simulink model "rlDQNPFC2"  (R2022b)
settings: Solver=FixedStepAuto  StartTime=0.0  StopTime=Tf  FixedStep=0.001  RelTol=1e-3
StartFcn:
  | %scopes= find_system(bdroot,'BlockType','Scope');
  | %for i = 1:length(scopes)
  | %set_param(scopes{i},'Open','on');
  | %end
values from neighbouring files (symbols this model uses):
  amax_ego = 0.4    [DDPG_1.m]    (also in DQN4.m)
  amin_ego = -0.5    [DDPG_1.m]    (also in DQN4.m)
  Cf = 19000    [DDPG_1.m]    (also in DQN4.m)
  Cr = 33000    [DDPG_1.m]    (also in DQN4.m)
  D_default = 1.5    [DDPG_1.m]    (also in DQN4.m)
  e1_initial = -0.05    [DDPG_1.m]    (also in DQN4.m)
  e2_initial = 0.05    [DDPG_1.m]    (also in DQN4.m)
  Iz = 2875    [DDPG_1.m]    (also in DQN4.m)
  lf = 1.4    [DDPG_1.m]    (also in DQN4.m)
  lr = 1.6    [DDPG_1.m]    (also in DQN4.m)
  m = 1600    [DDPG_1.m]    (also in DQN4.m)
  t_gap = 1.4    [DDPG_1.m]    (also in DQN4.m)
  target = 1    [DDPG_1.m]    (also in DQN4.m = 3)
  tau = 0.5    [DDPG_1.m]    (also in DQN4.m)
  Ts = 0.1    [DDPG_1.m]    (also in DQN4.m)
  umax_ego = 0.2618    [DDPG_1.m]    (also in DQN4.m)
  umin_ego = -0.2618    [DDPG_1.m]    (also in DQN4.m)
  v0_FV1 = 0.5    [DDPG_1.m]    (also in DQN4.m)
  v0_FV2 = 0.5    [DDPG_1.m]    (also in DQN4.m)
  v0_LV = 0.9    [DDPG_1.m]    (also in DQN4.m)
  v_set = 1.5    [DDPG_1.m]    (also in DQN4.m)
  x0_FV1 = 1.5    [DDPG_1.m]    (also in DQN4.m)
  x0_FV2 = 0    [DDPG_1.m]    (also in DQN4.m)
  x0_LV = 3    [DDPG_1.m]    (also in DQN4.m)
undefined symbols (not defined in the file or in its folder): DiscIntNeverNeededParam
libraries: simulink x13, rllib x4
settings Model: Creator=The MathWorks, Inc.  LastModifiedBy=Lenovo
settings SolverCC: AlgebraicLoopSolver=TrustRegion
settings DataIOCC: SaveOutput=off  SignalLogging=off  DSMLogging=off  SaveTime=off  ReturnWorkspaceOutputs=off
settings DebuggingCC: ParameterPrecisionLossMsg=none  UnconnectedInputMsg=warning  UnconnectedOutputMsg=warning  UnconnectedLineMsg=warning  SFMachineParentedDataDiag=warning  ArithmeticOperatorsInVariantConditions=warning
settings ModelReferenceCC: EnableRefExpFcnMdlSchedulingChecks=on
settings SFSimCC: SimUseLocalCustomCode=off
settings RTWCC: RTWUseLocalCustomCode=off

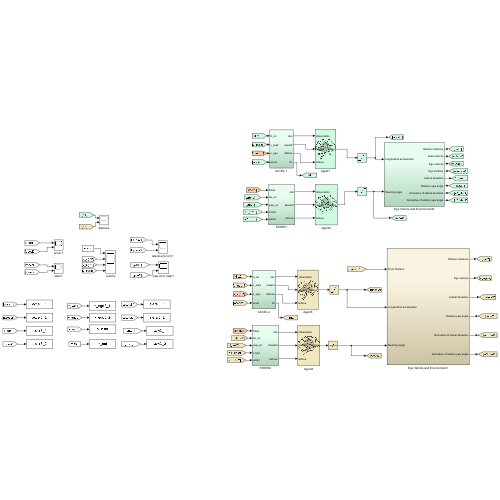
[thumbnail: Simulink's stored preview of the top-level diagram]
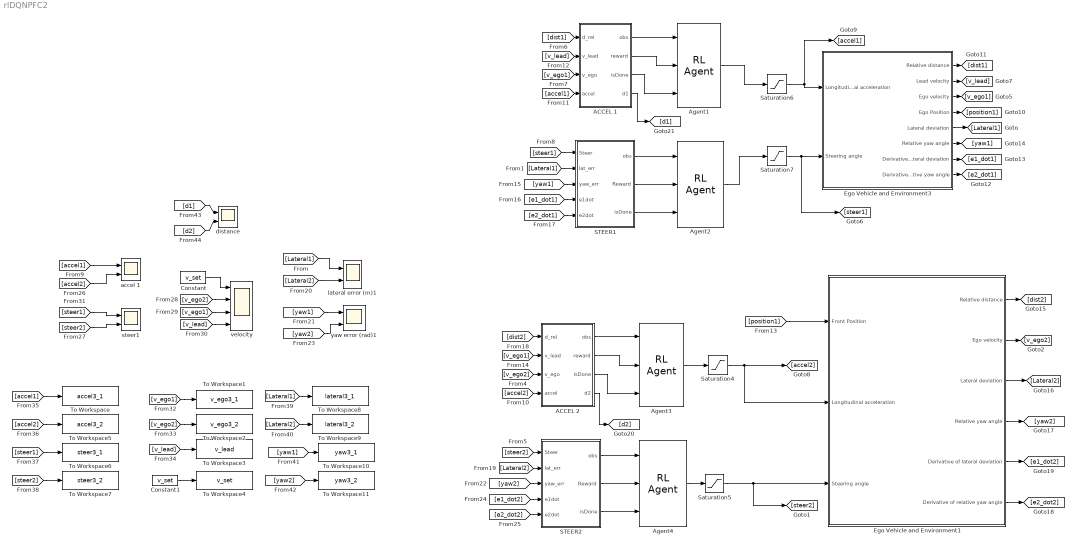
== system rlDQNPFC2 ==
  ACCEL 1 : Subsystem
  ACCEL 2 : Subsystem
  Agent1 : rllib/RL Agent  Agent=agent1  ExternalActionAsInput=off  ProvideLastAction=off  ProvideCumRwd=off  TreatAsDirectFeedthrough=on  UseStrictObservationDataTypes=off
  Agent2 : rllib/RL Agent  Agent=agent2  ExternalActionAsInput=off  ProvideLastAction=off  ProvideCumRwd=off  TreatAsDirectFeedthrough=on  UseStrictObservationDataTypes=off
  Agent3 : rllib/RL Agent  Agent=agent3  ExternalActionAsInput=off  ProvideLastAction=off  ProvideCumRwd=off  TreatAsDirectFeedthrough=on  UseStrictObservationDataTypes=off
  Agent4 : rllib/RL Agent  Agent=agent4  ExternalActionAsInput=off  ProvideLastAction=off  ProvideCumRwd=off  TreatAsDirectFeedthrough=on  UseStrictObservationDataTypes=off
  Constant : Constant  Value=v_set
  Constant1 : Constant  Value=v_set
  Ego Vehicle and Environment1 : Subsystem
  Ego Vehicle and Environment3 : Subsystem
  STEER1 : Subsystem
  STEER2 : Subsystem
  Saturation4 : Saturate  UpperLimit=amax_ego  LowerLimit=amin_ego
  Saturation5 : Saturate  UpperLimit=umax_ego  LowerLimit=umin_ego
  Saturation6 : Saturate  UpperLimit=amax_ego  LowerLimit=amin_ego
  Saturation7 : Saturate  UpperLimit=umax_ego  LowerLimit=umin_ego
  To Workspace : ToWorkspace  VariableName=accel3_1  SampleTime=-1
      settings: Save2DSignal=2-D array (concatenate along first dimension)
  To Workspace1 : ToWorkspace  VariableName=v_ego3_1  SampleTime=-1
      settings: Save2DSignal=2-D array (concatenate along first dimension)
  To Workspace10 : ToWorkspace  VariableName=yaw3_1  SampleTime=-1
      settings: Save2DSignal=2-D array (concatenate along first dimension)
  To Workspace11 : ToWorkspace  VariableName=yaw3_2  SampleTime=-1
      settings: Save2DSignal=2-D array (concatenate along first dimension)
  To Workspace2 : ToWorkspace  VariableName=v_ego3_2  SampleTime=-1
      settings: Save2DSignal=2-D array (concatenate along first dimension)
  To Workspace3 : ToWorkspace  VariableName=v_lead  SampleTime=-1
      settings: Save2DSignal=2-D array (concatenate along first dimension)
  To Workspace4 : ToWorkspace  VariableName=v_set  SampleTime=-1
      settings: Save2DSignal=2-D array (concatenate along first dimension)
  To Workspace5 : ToWorkspace  VariableName=accel3_2  SampleTime=-1
      settings: Save2DSignal=2-D array (concatenate along first dimension)
  To Workspace6 : ToWorkspace  VariableName=steer3_1  SampleTime=-1
      settings: Save2DSignal=2-D array (concatenate along first dimension)
  To Workspace7 : ToWorkspace  VariableName=steer3_2  SampleTime=-1
      settings: Save2DSignal=2-D array (concatenate along first dimension)
  To Workspace8 : ToWorkspace  VariableName=lateral3_1  SampleTime=-1
      settings: Save2DSignal=2-D array (concatenate along first dimension)
  To Workspace9 : ToWorkspace  VariableName=lateral3_2  SampleTime=-1
      settings: Save2DSignal=2-D array (concatenate along first dimension)
  accel 1 : Scope  NumInputPorts=2
  distance : Scope  NumInputPorts=2
  lateral error (m)1 : Scope  NumInputPorts=2
  steer1 : Scope  NumInputPorts=2
  velocity : Scope  NumInputPorts=4
  yaw error (rad)1 : Scope  NumInputPorts=2
  wires:
  [steer1] -> steer1/1
  Ego Vehicle and Environment1/2(Ego velocity) -> [v_ego2]
  [Lateral2] -> STEER2/2(lat_err)
  [v_ego1] -> velocity/3
  Agent3/1 -> Saturation4/1
  Constant/1 -> velocity/1
  [steer2] -> steer1/2
  [accel2] -> accel 1/2
  [accel1] -> accel 1/1
  [yaw2] -> yaw error (rad)1/2
  Ego Vehicle and Environment1/5(Derivative of lateral deviation) -> [e1_dot2]
  Ego Vehicle and Environment1/4(Relative yaw angle) -> [yaw2]
  [yaw2] -> STEER2/3(yaw_err)
  Saturation4/1 -> Ego Vehicle and Environment1/2(Longitudinal acceleration), [accel2]
  [yaw1] -> yaw error (rad)1/1
  [dist2] -> ACCEL 2/1(d_rel)
  [position1] -> Ego Vehicle and Environment1/1(Front Position)
  [v_ego2] -> ACCEL 2/3(v_ego)
  [Lateral2] -> lateral error (m)1/2
  Ego Vehicle and Environment1/6(Derivative of relative yaw angle) -> [e2_dot2]
  [v_ego1] -> ACCEL 2/2(v_lead)
  [steer2] -> STEER2/1(Steer)
  ACCEL 2/1(obs) -> Agent3/1
  ACCEL 2/3(isDone) -> Agent3/3
  STEER2/2(Reward) -> Agent4/2
  STEER2/1(obs) -> Agent4/1
  [v_lead] -> velocity/4
  Ego Vehicle and Environment1/1(Relative distance) -> [dist2]
  [Lateral1] -> lateral error (m)1/1
  [e2_dot2] -> STEER2/5(e2dot)
  Saturation5/1 -> [steer2], Ego Vehicle and Environment1/3(Steering angle)
  STEER2/3(isDone) -> Agent4/3
  Agent4/1 -> Saturation5/1
  Ego Vehicle and Environment1/3(Lateral deviation) -> [Lateral2]
  [accel2] -> ACCEL 2/4(accel)
  [v_ego2] -> velocity/2
  [e1_dot2] -> STEER2/4("e1dot ")
  ACCEL 2/2(reward) -> Agent3/2
  [v_ego1] -> To Workspace1/1
  [v_ego2] -> To Workspace2/1
  [v_lead] -> To Workspace3/1
  Constant1/1 -> To Workspace4/1
  [accel1] -> To Workspace/1
  [accel2] -> To Workspace5/1
  [steer1] -> To Workspace6/1
  [steer2] -> To Workspace7/1
  [Lateral1] -> To Workspace8/1
  [Lateral2] -> To Workspace9/1
  [yaw1] -> To Workspace10/1
  [yaw2] -> To Workspace11/1
  [yaw1] -> STEER1/3(yaw_err)
  [steer1] -> STEER1/1(Steer)
  Ego Vehicle and Environment3/5(Lateral deviation) -> [Lateral1]
  Ego Vehicle and Environment3/6(Relative yaw angle) -> [yaw1]
  Ego Vehicle and Environment3/2(Lead velocity) -> [v_lead]
  [dist1] -> ACCEL 1/1(d_rel)
  Ego Vehicle and Environment3/8(Derivative of relative yaw angle) -> [e2_dot1]
  Ego Vehicle and Environment3/4(Ego Position) -> [position1]
  Saturation7/1 -> Ego Vehicle and Environment3/2(Steering angle), [steer1]
  STEER1/3(isDone) -> Agent2/3
  ACCEL 1/2(reward) -> Agent1/2
  [e2_dot1] -> STEER1/5(e2dot)
  Agent2/1 -> Saturation7/1
  STEER1/2(Reward) -> Agent2/2
  [Lateral1] -> STEER1/2(lat_err)
  [accel1] -> ACCEL 1/4(accel)
  ACCEL 1/3(isDone) -> Agent1/3
  Ego Vehicle and Environment3/3(Ego velocity) -> [v_ego1]
  [e1_dot1] -> STEER1/4("e1dot ")
  Saturation6/1 -> Ego Vehicle and Environment3/1(Longitudinal acceleration), [accel1]
  Ego Vehicle and Environment3/1(Relative distance) -> [dist1]
  STEER1/1(obs) -> Agent2/1
  [v_ego1] -> ACCEL 1/3(v_ego)
  Ego Vehicle and Environment3/7(Derivative of lateral deviation) -> [e1_dot1]
  ACCEL 1/1(obs) -> Agent1/1
  Agent1/1 -> Saturation6/1
  [v_lead] -> ACCEL 1/2(v_lead)
  ACCEL 2/4(d2) -> [d2]
  ACCEL 1/4(d1) -> [d1]
  [d1] -> distance/1
  [d2] -> distance/2

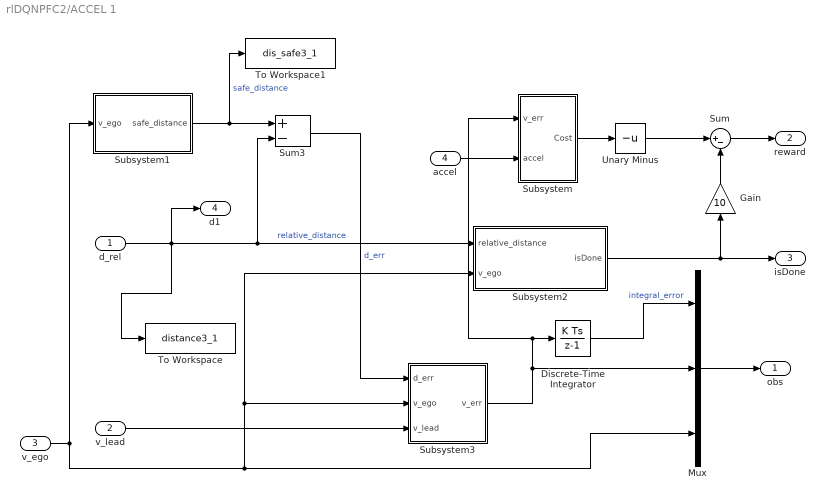
== system rlDQNPFC2/ACCEL 1 ==
  d_rel : Inport
  v_lead : Inport  Port=2
  v_ego : Inport  Port=3
  accel : Inport  Port=4
  Discrete-Time Integrator : DiscreteIntegrator  SampleTime=-1  ICPrevOutput=DiscIntNeverNeededParam  ICPrevScaledInput=DiscIntNeverNeededParam
  Gain : Gain  Gain=10
  Mux : Mux  Inputs=3
  Subsystem : Subsystem
  Subsystem1 : Subsystem
  Subsystem2 : Subsystem
  Subsystem3 : Subsystem
  Sum : Sum  Inputs=|+-
  Sum3 : Sum  Inputs=+-
  To Workspace : ToWorkspace  VariableName=distance3_1  SampleTime=-1
      settings: Save2DSignal=2-D array (concatenate along first dimension)
  To Workspace1 : ToWorkspace  VariableName=dis_safe3_1  SampleTime=-1
      settings: Save2DSignal=2-D array (concatenate along first dimension)
  Unary Minus : UnaryMinus
  obs : Outport  VectorParamsAs1DForOutWhenUnconnected=off
  reward : Outport  Port=2  VectorParamsAs1DForOutWhenUnconnected=off
  isDone : Outport  Port=3  VectorParamsAs1DForOutWhenUnconnected=off
  d1 : Outport  Port=4  VectorParamsAs1DForOutWhenUnconnected=off
  wires:
  v_lead/1 -> Subsystem3/3(v_lead)
  Discrete-Time Integrator/1 -> Mux/1  "integral_error"
  Mux/1 -> obs/1
  v_ego/1 -> Subsystem3/2(v_ego), Subsystem2/2(v_ego), Mux/3, Subsystem1/1(v_ego)
  d_rel/1 -> d1/1, To Workspace/1, Sum3/2, Subsystem2/1(relative_distance)  "relative_distance"
  Subsystem/1(Cost) -> Unary Minus/1
  Sum3/1 -> Subsystem3/1(d_err)  "d_err"
  Subsystem1/1(safe_distance) -> To Workspace1/1, Sum3/1  "safe_distance"
  accel/1 -> Subsystem/2(accel)
  Subsystem3/1(v_err) -> Mux/2, Subsystem/1(v_err), Discrete-Time Integrator/1
  Subsystem2/1(isDone) -> isDone/1, Gain/1
  Unary Minus/1 -> Sum/1
  Gain/1 -> Sum/2
  Sum/1 -> reward/1

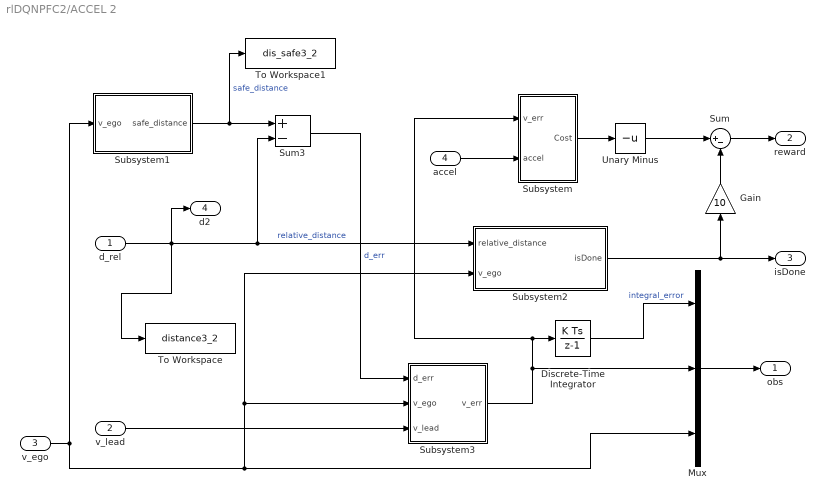
== system rlDQNPFC2/ACCEL 2 ==
  d_rel : Inport
  v_lead : Inport  Port=2
  v_ego : Inport  Port=3
  accel : Inport  Port=4
  Discrete-Time Integrator : DiscreteIntegrator  SampleTime=-1  ICPrevOutput=DiscIntNeverNeededParam  ICPrevScaledInput=DiscIntNeverNeededParam
  Gain : Gain  Gain=10
  Mux : Mux  Inputs=3
  Subsystem : Subsystem
  Subsystem1 : Subsystem
  Subsystem2 : Subsystem
  Subsystem3 : Subsystem
  Sum : Sum  Inputs=|+-
  Sum3 : Sum  Inputs=+-
  To Workspace : ToWorkspace  VariableName=distance3_2  SampleTime=-1
      settings: Save2DSignal=2-D array (concatenate along first dimension)
  To Workspace1 : ToWorkspace  VariableName=dis_safe3_2  SampleTime=-1
      settings: Save2DSignal=2-D array (concatenate along first dimension)
  Unary Minus : UnaryMinus
  obs : Outport  VectorParamsAs1DForOutWhenUnconnected=off
  reward : Outport  Port=2  VectorParamsAs1DForOutWhenUnconnected=off
  isDone : Outport  Port=3  VectorParamsAs1DForOutWhenUnconnected=off
  d2 : Outport  Port=4  VectorParamsAs1DForOutWhenUnconnected=off
  wires:
  Sum/1 -> reward/1
  Gain/1 -> Sum/2
  Unary Minus/1 -> Sum/1
  Subsystem2/1(isDone) -> Gain/1, isDone/1
  Subsystem3/1(v_err) -> Discrete-Time Integrator/1, Subsystem/1(v_err), Mux/2
  accel/1 -> Subsystem/2(accel)
  Subsystem1/1(safe_distance) -> Sum3/1, To Workspace1/1  "safe_distance"
  Sum3/1 -> Subsystem3/1(d_err)  "d_err"
  Subsystem/1(Cost) -> Unary Minus/1
  d_rel/1 -> d2/1, Subsystem2/1(relative_distance), Sum3/2, To Workspace/1  "relative_distance"
  v_ego/1 -> Subsystem1/1(v_ego), Mux/3, Subsystem2/2(v_ego), Subsystem3/2(v_ego)
  Mux/1 -> obs/1
  Discrete-Time Integrator/1 -> Mux/1  "integral_error"
  v_lead/1 -> Subsystem3/3(v_lead)

== system rlDQNPFC2/Ego Vehicle and Environment1 ==
  Front Position : Inport
  Longitudinal acceleration : Inport  Port=2
  Steering angle : Inport  Port=3
  Ego sensor : Subsystem
  Ego vehicle : Subsystem
  Initial ego position : Constant  Value=x0_FV2
  Initial lateral deviation : Constant  Value=e1_initial
  Initial relative yaw angle : Constant  Value=e2_initial
  Sum3 : Sum  Inputs=+-
  curvature1 : Subsystem
  Relative distance : Outport  VectorParamsAs1DForOutWhenUnconnected=off
  Ego velocity : Outport  Port=2  VectorParamsAs1DForOutWhenUnconnected=off
  Lateral deviation : Outport  Port=3  VectorParamsAs1DForOutWhenUnconnected=off
  Relative yaw angle : Outport  Port=4  VectorParamsAs1DForOutWhenUnconnected=off
  Derivative of lateral deviation : Outport  Port=5  VectorParamsAs1DForOutWhenUnconnected=off
  Derivative of relative yaw angle : Outport  Port=6  VectorParamsAs1DForOutWhenUnconnected=off
  wires:
  Ego vehicle/3(Lateral Velocity) -> Ego sensor/2(Lateral velocity)
  Ego vehicle/4(Yaw Rate) -> Ego sensor/3(Yaw rate)
  Longitudinal acceleration/1 -> Ego vehicle/1(Acceleration)  "acceleration"
  Ego sensor/1(Lateral deviation) -> Lateral deviation/1
  Ego vehicle/2(Longitudinal Velocity) -> Ego velocity/1, Ego sensor/1(Longitudinal velocity)
  Steering angle/1 -> Ego vehicle/2(Steering)  "steering"
  Ego sensor/2(Relative yaw angle) -> Relative yaw angle/1
  Initial lateral deviation/1 -> Ego sensor/6(Initial lateral deviation)
  Initial ego position/1 -> Ego vehicle/3(Initial position)
  curvature1/1(curvature) -> Ego sensor/4(Curvature)
  Initial relative yaw angle/1 -> Ego sensor/5(Initial relative yaw angle)
  Front Position/1 -> Sum3/1
  Ego vehicle/1(Position) -> curvature1/1(position), Sum3/2
  Sum3/1 -> Relative distance/1
  Ego sensor/3(e1_dot) -> Derivative of lateral deviation/1
  Ego sensor/4(e2_dot) -> Derivative of relative yaw angle/1

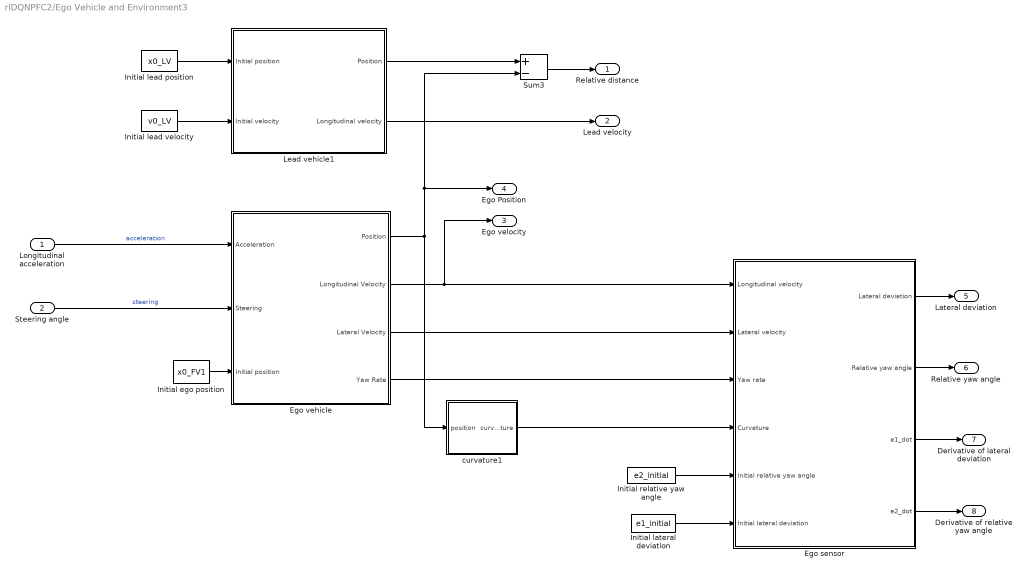
== system rlDQNPFC2/Ego Vehicle and Environment3 ==
  Longitudinal acceleration : Inport
  Steering angle : Inport  Port=2
  Ego sensor : Subsystem
  Ego vehicle : Subsystem
  Initial ego position : Constant  Value=x0_FV1
  Initial lateral deviation : Constant  Value=e1_initial
  Initial lead position : Constant  Value=x0_LV
  Initial lead velocity : Constant  Value=v0_LV
  Initial relative yaw angle : Constant  Value=e2_initial
  Lead vehicle1 : Subsystem
  Sum3 : Sum  Inputs=+-
  curvature1 : Subsystem
  Relative distance : Outport  VectorParamsAs1DForOutWhenUnconnected=off
  Lead velocity : Outport  Port=2  VectorParamsAs1DForOutWhenUnconnected=off
  Ego velocity : Outport  Port=3  VectorParamsAs1DForOutWhenUnconnected=off
  Ego Position : Outport  Port=4
  Lateral deviation : Outport  Port=5  VectorParamsAs1DForOutWhenUnconnected=off
  Relative yaw angle : Outport  Port=6  VectorParamsAs1DForOutWhenUnconnected=off
  Derivative of lateral deviation : Outport  Port=7  VectorParamsAs1DForOutWhenUnconnected=off
  Derivative of relative yaw angle : Outport  Port=8  VectorParamsAs1DForOutWhenUnconnected=off
  wires:
  Ego vehicle/3(Lateral Velocity) -> Ego sensor/2(Lateral velocity)
  Ego vehicle/4(Yaw Rate) -> Ego sensor/3(Yaw rate)
  Longitudinal acceleration/1 -> Ego vehicle/1(Acceleration)  "acceleration"
  Ego sensor/1(Lateral deviation) -> Lateral deviation/1
  Ego vehicle/2(Longitudinal Velocity) -> Ego velocity/1, Ego sensor/1(Longitudinal velocity)
  Steering angle/1 -> Ego vehicle/2(Steering)  "steering"
  Ego sensor/2(Relative yaw angle) -> Relative yaw angle/1
  Initial lateral deviation/1 -> Ego sensor/6(Initial lateral deviation)
  Initial ego position/1 -> Ego vehicle/3(Initial position)
  curvature1/1(curvature) -> Ego sensor/4(Curvature)
  Initial relative yaw angle/1 -> Ego sensor/5(Initial relative yaw angle)
  Initial lead velocity/1 -> Lead vehicle1/2(Initial velocity)
  Initial lead position/1 -> Lead vehicle1/1(Initial position)
  Lead vehicle1/1(Position) -> Sum3/1
  Ego vehicle/1(Position) -> curvature1/1(position), Ego Position/1, Sum3/2
  Sum3/1 -> Relative distance/1
  Lead vehicle1/2(Longitudinal velocity) -> Lead velocity/1
  Ego sensor/3(e1_dot) -> Derivative of lateral deviation/1
  Ego sensor/4(e2_dot) -> Derivative of relative yaw angle/1

== system rlDQNPFC2/STEER1 ==
  Steer : Inport
  lat_err : Inport  Port=2
  yaw_err : Inport  Port=3
  "e1dot " : Inport  Port=4
  e2dot : Inport  Port=5
  Abs : Abs  SaturateOnIntegerOverflow=off
  Compare To Constant : simulink/Logic and Bit Operations/Compare To Constant  relop=>  const=1  OutDataTypeStr=boolean
  Gain : Gain  Gain=10
  Subsystem : Subsystem
  Subsystem1 : Subsystem
  Sum : Sum  Inputs=-+|
  Unary Minus : UnaryMinus
  obs : Outport  VectorParamsAs1DForOutWhenUnconnected=off
  Reward : Outport  Port=2  VectorParamsAs1DForOutWhenUnconnected=off
  isDone : Outport  Port=3  VectorParamsAs1DForOutWhenUnconnected=off
  wires:
  Subsystem/1(Cost) -> Unary Minus/1
  lat_err/1 -> Subsystem1/1(e1), Subsystem/2(e1), Abs/1
  yaw_err/1 -> Subsystem1/2(e2)
  Abs/1 -> Compare To Constant/1
  Subsystem1/1(obs) -> obs/1
  "e1dot "/1 -> Subsystem1/3(e1dot)
  e2dot/1 -> Subsystem1/4(e2dot)
  Steer/1 -> Subsystem/1(steer)
  Compare To Constant/1 -> isDone/1, Gain/1
  Gain/1 -> Sum/1
  Sum/1 -> Reward/1
  Unary Minus/1 -> Sum/2

== system rlDQNPFC2/STEER2 ==
  Steer : Inport
  lat_err : Inport  Port=2
  yaw_err : Inport  Port=3
  "e1dot " : Inport  Port=4
  e2dot : Inport  Port=5
  Abs : Abs  SaturateOnIntegerOverflow=off
  Compare To Constant : simulink/Logic and Bit Operations/Compare To Constant  relop=>  const=1  OutDataTypeStr=boolean
  Gain : Gain  Gain=10
  Subsystem : Subsystem
  Subsystem1 : Subsystem
  Sum : Sum  Inputs=-+|
  Unary Minus : UnaryMinus
  obs : Outport  VectorParamsAs1DForOutWhenUnconnected=off
  Reward : Outport  Port=2  VectorParamsAs1DForOutWhenUnconnected=off
  isDone : Outport  Port=3  VectorParamsAs1DForOutWhenUnconnected=off
  wires:
  Unary Minus/1 -> Sum/2
  Sum/1 -> Reward/1
  Gain/1 -> Sum/1
  Compare To Constant/1 -> Gain/1, isDone/1
  Steer/1 -> Subsystem/1(steer)
  e2dot/1 -> Subsystem1/4(e2dot)
  "e1dot "/1 -> Subsystem1/3(e1dot)
  Subsystem1/1(obs) -> obs/1
  Abs/1 -> Compare To Constant/1
  yaw_err/1 -> Subsystem1/2(e2)
  lat_err/1 -> Abs/1, Subsystem/2(e1), Subsystem1/1(e1)
  Subsystem/1(Cost) -> Unary Minus/1

== system rlDQNPFC2/ACCEL 1/Subsystem ==
  v_err : Inport
  accel : Inport  Port=2
  Compare To Constant : simulink/Logic and Bit Operations/Compare To Constant  relop=<  const=0.09  OutDataTypeStr=boolean
  Gain1 : Gain  Gain=0.1
  Gain2 : Gain  Gain=0.01
  Gain3 : Gain
  Math Function2 : Math  Operator=square  SignedPower=on
  Square : Math  Operator=square  SignedPower=on
  Sum : Sum  Inputs=++-
  Unit Delay : UnitDelay  SampleTime=-1  HasFrameUpgradeWarning=on
  Cost : Outport  VectorParamsAs1DForOutWhenUnconnected=off
  wires:
  v_err/1 -> Square/1
  Math Function2/1 -> Gain1/1
  accel/1 -> Unit Delay/1
  Sum/1 -> Cost/1
  Square/1 -> Compare To Constant/1, Gain2/1
  Unit Delay/1 -> Math Function2/1
  Gain2/1 -> Sum/1
  Gain1/1 -> Sum/2
  Compare To Constant/1 -> Gain3/1
  Gain3/1 -> Sum/3

== system rlDQNPFC2/ACCEL 1/Subsystem1 ==
  v_ego : Inport
  Default Spacing : Constant  Value=D_default  SampleTime=Ts
  Product : Product
  Sum2 : Sum
  Time Gap : Constant  Value=t_gap  SampleTime=Ts
  safe_distance : Outport  VectorParamsAs1DForOutWhenUnconnected=off
  wires:
  Sum2/1 -> safe_distance/1
  Product/1 -> Sum2/2
  Time Gap/1 -> Product/2
  Default Spacing/1 -> Sum2/1
  v_ego/1 -> Product/1

== system rlDQNPFC2/ACCEL 1/Subsystem2 ==
  relative_distance : Inport
  v_ego : Inport  Port=2
  Logical Operator : Logic  Operator=OR  AllPortsSameDT=off  OutDataTypeStr=boolean
  Relative Distance : simulink/Logic and Bit Operations/Compare To Constant  relop=<  const=0  OutDataTypeStr=boolean
  Velocity : simulink/Logic and Bit Operations/Compare To Constant  relop=<  const=0.05  OutDataTypeStr=boolean
  isDone : Outport  VectorParamsAs1DForOutWhenUnconnected=off
  wires:
  Velocity/1 -> Logical Operator/2
  Relative Distance/1 -> Logical Operator/1
  relative_distance/1 -> Relative Distance/1
  Logical Operator/1 -> isDone/1
  v_ego/1 -> Velocity/1

== system rlDQNPFC2/ACCEL 1/Subsystem3 ==
  d_err : Inport
  v_ego : Inport  Port=2
  v_lead : Inport  Port=3
  Constant : Constant  Value=v_set
  Min : MinMax  Inputs=2
  Sum1 : Sum  Inputs=+-
  Switch : Switch  Criteria=u2 > Threshold  SaturateOnIntegerOverflow=off  InputSameDT=off
  v_err : Outport  VectorParamsAs1DForOutWhenUnconnected=off
  wires:
  Sum1/1 -> v_err/1
  v_ego/1 -> Sum1/2
  Switch/1 -> Sum1/1  "v_ref"
  d_err/1 -> Switch/2
  Constant/1 -> Min/2, Switch/3
  Min/1 -> Switch/1
  v_lead/1 -> Min/1

== system rlDQNPFC2/ACCEL 2/Subsystem ==
  v_err : Inport
  accel : Inport  Port=2
  Compare To Constant : simulink/Logic and Bit Operations/Compare To Constant  relop=<  const=0.09  OutDataTypeStr=boolean
  Gain1 : Gain  Gain=0.1
  Gain2 : Gain  Gain=0.01
  Gain3 : Gain
  Math Function2 : Math  Operator=square  SignedPower=on
  Square : Math  Operator=square  SignedPower=on
  Sum : Sum  Inputs=++-
  Unit Delay : UnitDelay  SampleTime=-1  HasFrameUpgradeWarning=on
  Cost : Outport  VectorParamsAs1DForOutWhenUnconnected=off
  wires:
  Gain3/1 -> Sum/3
  Compare To Constant/1 -> Gain3/1
  Gain1/1 -> Sum/2
  Gain2/1 -> Sum/1
  Unit Delay/1 -> Math Function2/1
  Square/1 -> Gain2/1, Compare To Constant/1
  Sum/1 -> Cost/1
  accel/1 -> Unit Delay/1
  Math Function2/1 -> Gain1/1
  v_err/1 -> Square/1

== system rlDQNPFC2/ACCEL 2/Subsystem1 ==
  v_ego : Inport
  Default Spacing : Constant  Value=D_default  SampleTime=Ts
  Product : Product
  Sum2 : Sum
  Time Gap : Constant  Value=t_gap  SampleTime=Ts
  safe_distance : Outport  VectorParamsAs1DForOutWhenUnconnected=off
  wires:
  v_ego/1 -> Product/1
  Default Spacing/1 -> Sum2/1
  Time Gap/1 -> Product/2
  Product/1 -> Sum2/2
  Sum2/1 -> safe_distance/1

== system rlDQNPFC2/ACCEL 2/Subsystem2 ==
  relative_distance : Inport
  v_ego : Inport  Port=2
  Logical Operator : Logic  Operator=OR  AllPortsSameDT=off  OutDataTypeStr=boolean
  Relative Distance : simulink/Logic and Bit Operations/Compare To Constant  relop=<  const=0  OutDataTypeStr=boolean
  Velocity : simulink/Logic and Bit Operations/Compare To Constant  relop=<  const=0.05  OutDataTypeStr=boolean
  isDone : Outport  VectorParamsAs1DForOutWhenUnconnected=off
  wires:
  v_ego/1 -> Velocity/1
  Logical Operator/1 -> isDone/1
  relative_distance/1 -> Relative Distance/1
  Relative Distance/1 -> Logical Operator/1
  Velocity/1 -> Logical Operator/2

== system rlDQNPFC2/ACCEL 2/Subsystem3 ==
  d_err : Inport
  v_ego : Inport  Port=2
  v_lead : Inport  Port=3
  Constant : Constant  Value=v_set
  Min : MinMax  Inputs=2
  Sum1 : Sum  Inputs=+-
  Switch : Switch  Criteria=u2 > Threshold  SaturateOnIntegerOverflow=off  InputSameDT=off
  v_err : Outport  VectorParamsAs1DForOutWhenUnconnected=off
  wires:
  v_lead/1 -> Min/1
  Min/1 -> Switch/1
  Constant/1 -> Switch/3, Min/2
  d_err/1 -> Switch/2
  Switch/1 -> Sum1/1  "v_ref"
  v_ego/1 -> Sum1/2
  Sum1/1 -> v_err/1

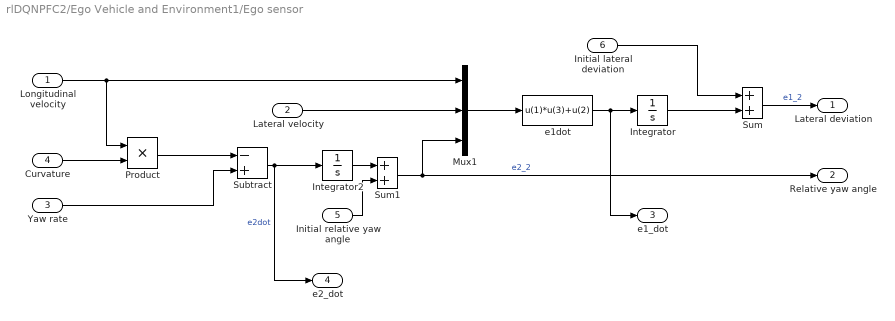
== system rlDQNPFC2/Ego Vehicle and Environment1/Ego sensor ==
  Longitudinal velocity : Inport
  Lateral velocity : Inport  Port=2
  Yaw rate : Inport  Port=3
  Curvature : Inport  Port=4
  Initial relative yaw angle : Inport  Port=5
  Initial lateral deviation : Inport  Port=6
  Integrator : Integrator
  Integrator2 : Integrator
  Mux1 : Mux  Inputs=[1 1 1]
  Product : Product
  Subtract : Sum  Inputs=-+
  Sum : Sum
  Sum1 : Sum
  e1dot : Fcn  Expr=u(1)*u(3)+u(2)
  Lateral deviation : Outport  VectorParamsAs1DForOutWhenUnconnected=off
  Relative yaw angle : Outport  Port=2  VectorParamsAs1DForOutWhenUnconnected=off
  e1_dot : Outport  Port=3  VectorParamsAs1DForOutWhenUnconnected=off
  e2_dot : Outport  Port=4  VectorParamsAs1DForOutWhenUnconnected=off
  wires:
  Curvature/1 -> Product/2
  Sum1/1 -> Mux1/3, Relative yaw angle/1  "e2_2"
  Mux1/1 -> e1dot/1
  Initial lateral deviation/1 -> Sum/1
  e1dot/1 -> e1_dot/1, Integrator/1
  Integrator/1 -> Sum/2
  Longitudinal velocity/1 -> Product/1, Mux1/1
  Lateral velocity/1 -> Mux1/2
  Sum/1 -> Lateral deviation/1  "e1_2"
  Integrator2/1 -> Sum1/1
  Initial relative yaw angle/1 -> Sum1/2
  Product/1 -> Subtract/1
  Yaw rate/1 -> Subtract/2
  Subtract/1 -> e2_dot/1, Integrator2/1  "e2dot"

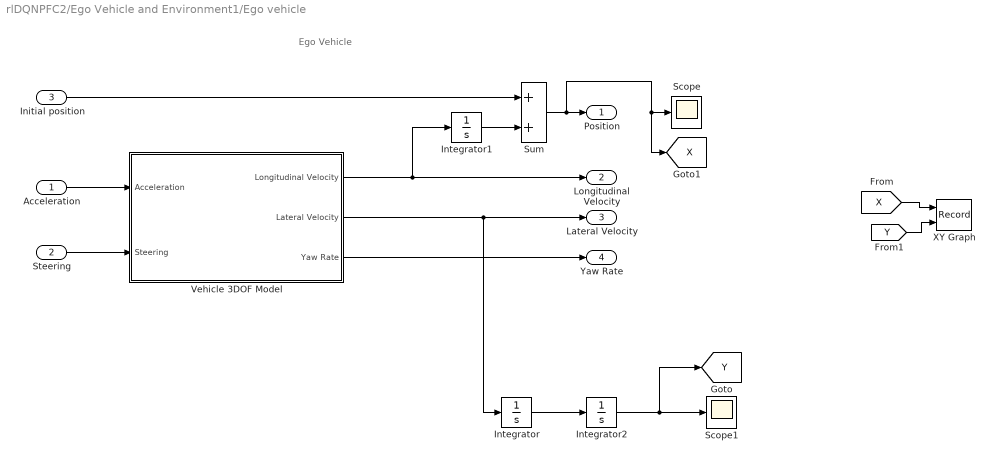
== system rlDQNPFC2/Ego Vehicle and Environment1/Ego vehicle ==
  note: Ego Vehicle
  Acceleration : Inport
  Steering : Inport  Port=2
  Initial position : Inport  Port=3
  Integrator : Integrator
  Integrator1 : Integrator
  Integrator2 : Integrator
  Scope : Scope
  Scope1 : Scope
  Sum : Sum
  Vehicle 3DOF Model : Subsystem
  XY Graph : Record  FileSettingsInternal="{\"entries\":[{\"content\":{\"excelSettings\":{\"content\":{},\"type\":\"Streamout.ExcelSettings\"}},\"type\":\"Streamout.FileSettingStorage\",\"uuid\":\"926f95c6-678a-42c3-81c2-7d91716961ee\"}],\"packageUris\":[\"http://schema.mathworks.com/mf0/streamout_blocks/R2020a\"],\"version\":\"1.0\"}"  Layout=[1 1]  SignalsInternal="{\"entries\":[{\"content\":{\"signals\":[{\"content\":{\"blockPath\":[\"rlDQNPFC2/Ego Vehicle and Environment1/Ego vehicle/XY Graph\"],\"channel\":[],\"dimensions\":[1],\"domain\":\"rlDQNPFC2/Ego Vehicle and Environment1/Ego vehicle/XY Graph\",\"lineColor\":\"#139fff\",\"plots\":[],\"port\":1,\"sid\":[],\"signalID\":2481,\"signalName\":\"From\"},\"type\":\"RecordBlkView.Signal\",\"uuid\":\"ba51d43c-8927-4175-b2ca-93bf3e4e2194\"},{\"content\":{\"blockPath\":[\"rlDQNPFC2/Ego Vehicle and Environment1/Ego vehicle/XY Graph\"],\"channel\":[],\"dimensions\":[1],\"domain\":\"rlDQNPFC2/Ego Vehicle and Environment1/Ego vehicle/XY Graph\",\"lineColor\":\"#ff6929\",\"plots\":[],\"port\":2,\"sid\":[],\"signalID\":2484,\"signalName\":\"From1\"},\"type\":\"RecordBlkView.Signal\",\"uuid\":\"ffd6dc64-998e-4497-b7fe-adbc949d6770\"}]},\"type\":\"RecordBlkView.InputSignals\",\"uuid\":\"4b290cac-6114-4463-9ac7-c2a0d02c0e46\"}],\"packageUris\":[\"http://schema.mathworks.com/mf0/streamout_blocks/R2020a\"],\"version\":\"1.0\"}"  CompatibilityTag=XY
  Position : Outport  VectorParamsAs1DForOutWhenUnconnected=off
  Longitudinal Velocity : Outport  Port=2  VectorParamsAs1DForOutWhenUnconnected=off
  Lateral Velocity : Outport  Port=3  VectorParamsAs1DForOutWhenUnconnected=off
  Yaw Rate : Outport  Port=4  VectorParamsAs1DForOutWhenUnconnected=off
  tag scope: X=global, Y=global
  wires:
  Integrator1/1 -> Sum/2
  Initial position/1 -> Sum/1
  Acceleration/1 -> Vehicle 3DOF Model/1(Acceleration)
  Steering/1 -> Vehicle 3DOF Model/2(Steering)
  Vehicle 3DOF Model/3(Yaw Rate) -> Yaw Rate/1
  Vehicle 3DOF Model/1(Longitudinal Velocity) -> Longitudinal Velocity/1, Integrator1/1
  Sum/1 -> [X], Scope/1, Position/1
  Vehicle 3DOF Model/2(Lateral Velocity) -> Integrator/1, Lateral Velocity/1
  Integrator/1 -> Integrator2/1
  Integrator2/1 -> [Y], Scope1/1
  [X] -> XY Graph/1
  [Y] -> XY Graph/2

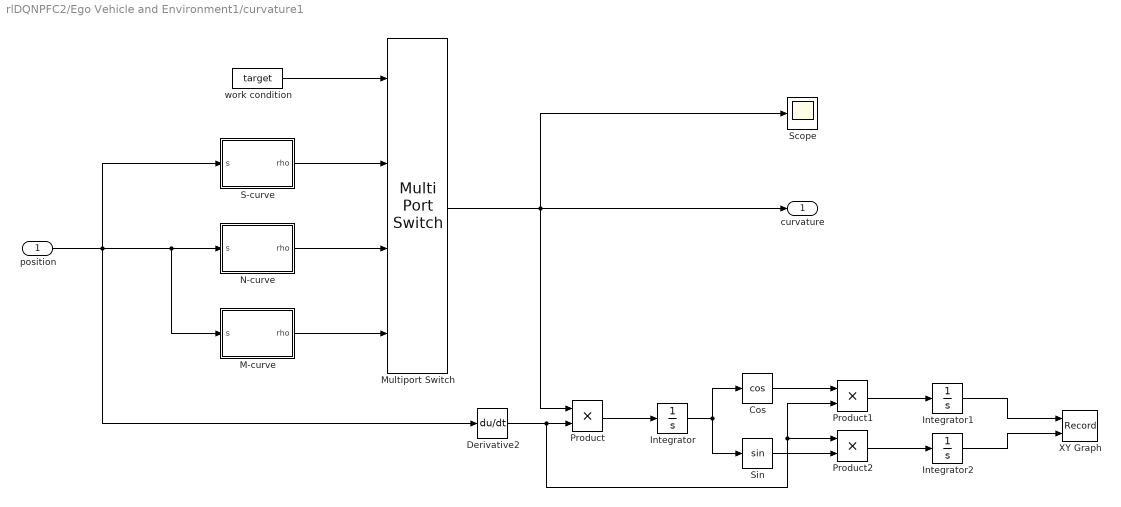
== system rlDQNPFC2/Ego Vehicle and Environment1/curvature1 ==
  position : Inport
  Cos : Trigonometry  Operator=cos
  Derivative2 : Derivative
  Integrator : Integrator
  Integrator1 : Integrator
  Integrator2 : Integrator
  M-curve : MATLAB Function  TreatAsAtomicUnit=on
  Multiport Switch : MultiPortSwitch  SaturateOnIntegerOverflow=off  InputSameDT=off
  N-curve : MATLAB Function  TreatAsAtomicUnit=on
  Product : Product
  Product1 : Product
  Product2 : Product
  S-curve : MATLAB Function  TreatAsAtomicUnit=on
  Scope : Scope
  Sin : Trigonometry
  XY Graph : Record  FileSettingsInternal="{\"entries\":[{\"content\":{\"excelSettings\":{\"content\":{},\"type\":\"Streamout.ExcelSettings\"}},\"type\":\"Streamout.FileSettingStorage\",\"uuid\":\"a88f7f64-6dc8-4fad-b474-f6daca30f32e\"}],\"packageUris\":[\"http://schema.mathworks.com/mf0/streamout_blocks/R2020a\"],\"version\":\"1.0\"}"  Layout=[1 1]  SignalsInternal="{\"entries\":[{\"content\":{\"signals\":[{\"content\":{\"blockPath\":[\"rlDQNPFC2/Ego Vehicle and Environment1/curvature1/XY Graph\"],\"channel\":[],\"dimensions\":[1],\"domain\":\"rlDQNPFC2/Ego Vehicle and Environment1/curvature1/XY Graph\",\"lineColor\":\"#b746ff\",\"plots\":[],\"port\":1,\"sid\":[],\"signalID\":2473,\"signalName\":\"Integrator1\"},\"type\":\"RecordBlkView.Signal\",\"uuid\":\"be24a98a-5aff-47ce-ad63-fb56a4aae694\"},{\"content\":{\"blockPath\":[\"rlDQNPFC2/Ego Vehicle and Environment1/curvature1/XY Graph\"],\"channel\":[],\"dimensions\":[1],\"domain\":\"rlDQNPFC2/Ego Vehicle and Environment1/curvature1/XY Graph\",\"lineColor\":\"#64d413\",\"plots\":[],\"port\":2,\"sid\":[],\"signalID\":2476,\"signalName\":\"Integrator2\"},\"type\":\"RecordBlkView.Signal\",\"uuid\":\"fdd17382-7340-4eb7-bf1d-fe8a0e01edb1\"}]},\"type\":\"RecordBlkView.InputSignals\",\"uuid\":\"159e895c-7bf5-4838-b84f-f7ecce4a2c9b\"}],\"packageUris\":[\"http://schema.mathworks.com/mf0/streamout_blocks/R2020a\"],\"version\":\"1.0\"}"  VisualizationBindings="{\"xyplotplugin\":{\"info\":[{\"series\":[],\"subplotID\":1}]}}"  CompatibilityTag=XY
  work condition : Constant  Value=target
  curvature : Outport
  wires:
  Integrator1/1 -> XY Graph/1
  Integrator2/1 -> XY Graph/2
  Integrator/1 -> Cos/1, Sin/1
  Derivative2/1 -> Product1/2, Product2/1, Product/2
  Product/1 -> Integrator/1
  Product2/1 -> Integrator2/1
  Sin/1 -> Product2/2
  Product1/1 -> Integrator1/1
  Cos/1 -> Product1/1
  position/1 -> S-curve/1(s), Derivative2/1, M-curve/1(s), N-curve/1(s)
  Multiport Switch/1 -> Product/1, curvature/1, Scope/1
  S-curve/1(rho) -> Multiport Switch/2
  N-curve/1(rho) -> Multiport Switch/3
  work condition/1 -> Multiport Switch/1
  M-curve/1(rho) -> Multiport Switch/4

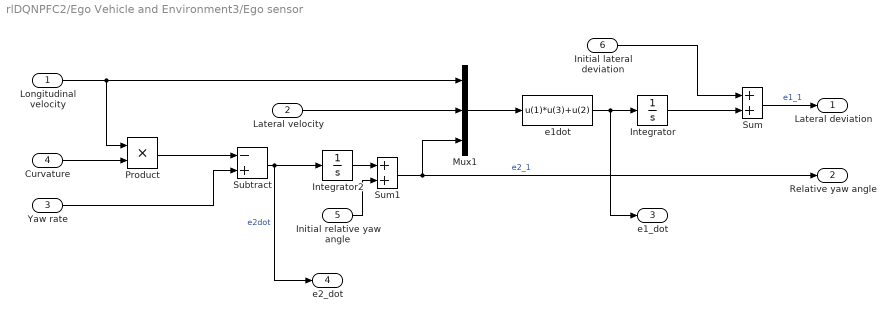
== system rlDQNPFC2/Ego Vehicle and Environment3/Ego sensor ==
  Longitudinal velocity : Inport
  Lateral velocity : Inport  Port=2
  Yaw rate : Inport  Port=3
  Curvature : Inport  Port=4
  Initial relative yaw angle : Inport  Port=5
  Initial lateral deviation : Inport  Port=6
  Integrator : Integrator
  Integrator2 : Integrator
  Mux1 : Mux  Inputs=[1 1 1]
  Product : Product
  Subtract : Sum  Inputs=-+
  Sum : Sum
  Sum1 : Sum
  e1dot : Fcn  Expr=u(1)*u(3)+u(2)
  Lateral deviation : Outport  VectorParamsAs1DForOutWhenUnconnected=off
  Relative yaw angle : Outport  Port=2  VectorParamsAs1DForOutWhenUnconnected=off
  e1_dot : Outport  Port=3  VectorParamsAs1DForOutWhenUnconnected=off
  e2_dot : Outport  Port=4  VectorParamsAs1DForOutWhenUnconnected=off
  wires:
  Curvature/1 -> Product/2
  Sum1/1 -> Mux1/3, Relative yaw angle/1  "e2_1"
  Mux1/1 -> e1dot/1
  Initial lateral deviation/1 -> Sum/1
  e1dot/1 -> e1_dot/1, Integrator/1
  Integrator/1 -> Sum/2
  Longitudinal velocity/1 -> Product/1, Mux1/1
  Lateral velocity/1 -> Mux1/2
  Sum/1 -> Lateral deviation/1  "e1_1"
  Integrator2/1 -> Sum1/1
  Initial relative yaw angle/1 -> Sum1/2
  Product/1 -> Subtract/1
  Yaw rate/1 -> Subtract/2
  Subtract/1 -> e2_dot/1, Integrator2/1  "e2dot"

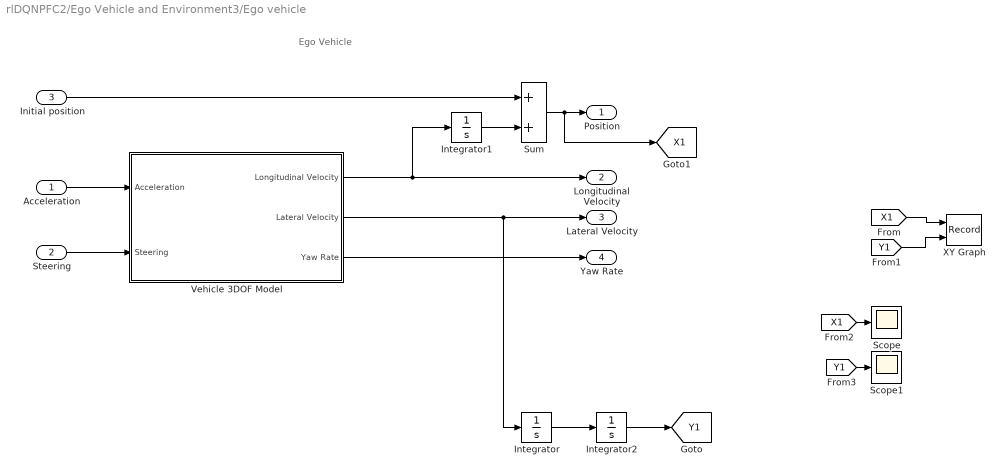
== system rlDQNPFC2/Ego Vehicle and Environment3/Ego vehicle ==
  note: Ego Vehicle
  Acceleration : Inport
  Steering : Inport  Port=2
  Initial position : Inport  Port=3
  Integrator : Integrator
  Integrator1 : Integrator
  Integrator2 : Integrator
  Scope : Scope
  Scope1 : Scope
  Sum : Sum
  Vehicle 3DOF Model : Subsystem
  XY Graph : Record  FileSettingsInternal="{\"entries\":[{\"content\":{\"excelSettings\":{\"content\":{},\"type\":\"Streamout.ExcelSettings\"}},\"type\":\"Streamout.FileSettingStorage\",\"uuid\":\"b77e72f0-3780-4628-8c22-82802707b8c2\"}],\"packageUris\":[\"http://schema.mathworks.com/mf0/streamout_blocks/R2020a\"],\"version\":\"1.0\"}"  Layout=[1 1]  SignalsInternal="{\"entries\":[{\"content\":{\"signals\":[{\"content\":{\"blockPath\":[\"rlDQNPFC2/Ego Vehicle and Environment3/Ego vehicle/XY Graph\"],\"channel\":[],\"dimensions\":[1],\"domain\":\"rlDQNPFC2/Ego Vehicle and Environment3/Ego vehicle/XY Graph\",\"lineColor\":\"#ff13a6\",\"plots\":[],\"port\":1,\"sid\":[],\"signalID\":2465,\"signalName\":\"From\"},\"type\":\"RecordBlkView.Signal\",\"uuid\":\"8eb38749-574b-4766-8d65-6162ff162a27\"},{\"content\":{\"blockPath\":[\"rlDQNPFC2/Ego Vehicle and Environment3/Ego vehicle/XY Graph\"],\"channel\":[],\"dimensions\":[1],\"domain\":\"rlDQNPFC2/Ego Vehicle and Environment3/Ego vehicle/XY Graph\",\"lineColor\":\"#fe330a\",\"plots\":[],\"port\":2,\"sid\":[],\"signalID\":2468,\"signalName\":\"From1\"},\"type\":\"RecordBlkView.Signal\",\"uuid\":\"504250fa-d97e-40d2-a22b-9ec899ac93c3\"}]},\"type\":\"RecordBlkView.InputSignals\",\"uuid\":\"abb257bf-f213-4b71-872b-4d0fb6c25c0d\"}],\"packageUris\":[\"http://schema.mathworks.com/mf0/streamout_blocks/R2020a\"],\"version\":\"1.0\"}"  VisualizationBindings="{\"sparklinesplugin\":{\"info\":[{\"bindingParametersList\":[],\"subplotID\":1}]}}"  CompatibilityTag=XY
  Position : Outport  VectorParamsAs1DForOutWhenUnconnected=off
  Longitudinal Velocity : Outport  Port=2  VectorParamsAs1DForOutWhenUnconnected=off
  Lateral Velocity : Outport  Port=3  VectorParamsAs1DForOutWhenUnconnected=off
  Yaw Rate : Outport  Port=4  VectorParamsAs1DForOutWhenUnconnected=off
  tag scope: X1=global, Y1=global
  wires:
  Integrator1/1 -> Sum/2
  Initial position/1 -> Sum/1
  Acceleration/1 -> Vehicle 3DOF Model/1(Acceleration)
  Steering/1 -> Vehicle 3DOF Model/2(Steering)
  Vehicle 3DOF Model/3(Yaw Rate) -> Yaw Rate/1
  Vehicle 3DOF Model/1(Longitudinal Velocity) -> Longitudinal Velocity/1, Integrator1/1
  Vehicle 3DOF Model/2(Lateral Velocity) -> Integrator/1, Lateral Velocity/1
  Sum/1 -> [X1], Position/1
  Integrator2/1 -> [Y1]
  Integrator/1 -> Integrator2/1
  [X1] -> XY Graph/1
  [Y1] -> XY Graph/2
  [X1] -> Scope/1
  [Y1] -> Scope1/1

== system rlDQNPFC2/Ego Vehicle and Environment3/Lead vehicle1 ==
  Initial position : Inport
  Initial velocity : Inport  Port=2
  Constant : Constant  Value=target
  Integrator : Integrator
  Integrator1 : Integrator
  Multiport Switch1 : MultiPortSwitch  SaturateOnIntegerOverflow=off  InputSameDT=off
  Sine1 : Sin  Amplitude=0.05  Frequency=2*pi/60  SampleTime=Ts
  Sum : Sum
  Sum1 : Sum
  Transfer Fcn : TransferFcn  Denominator=[0.6 1]
  a_LV : Scope
  ramp1 : Subsystem
  step1 : Subsystem
  Position : Outport  VectorParamsAs1DForOutWhenUnconnected=off
  Longitudinal velocity : Outport  Port=2  VectorParamsAs1DForOutWhenUnconnected=off
  wires:
  Transfer Fcn/1 -> Sum1/1
  Initial velocity/1 -> Sum1/2
  Sum/1 -> Position/1
  Integrator/1 -> Transfer Fcn/1
  Sum1/1 -> Integrator1/1, Longitudinal velocity/1
  Initial position/1 -> Sum/1
  Integrator1/1 -> Sum/2
  Sine1/1 -> Multiport Switch1/3  "a_LV"
  ramp1/1(Out1) -> Multiport Switch1/2
  step1/1(a_LV) -> Multiport Switch1/4
  Multiport Switch1/1 -> a_LV/1, Integrator/1  "a_LV"
  Constant/1 -> Multiport Switch1/1

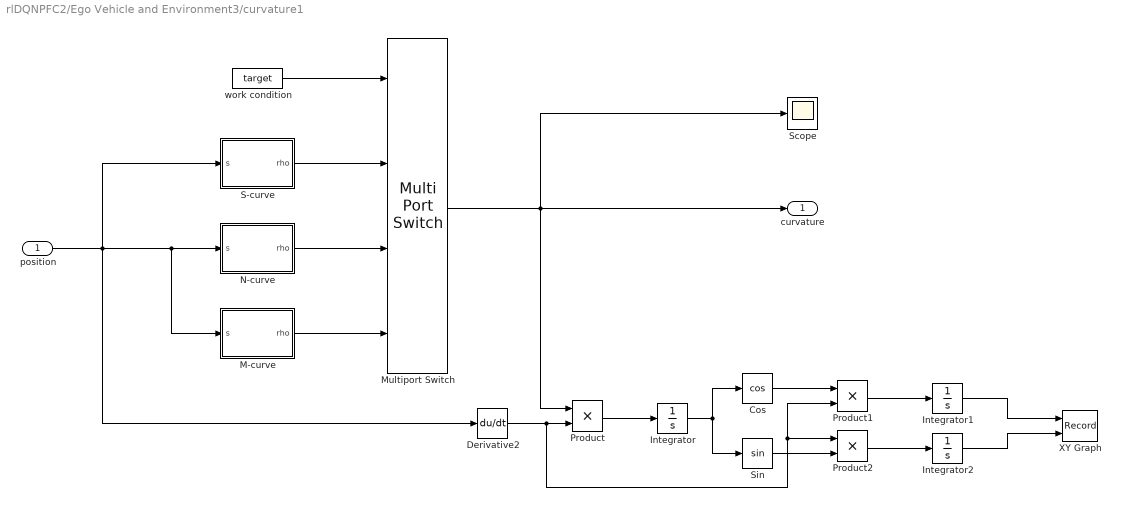
== system rlDQNPFC2/Ego Vehicle and Environment3/curvature1 ==
  position : Inport
  Cos : Trigonometry  Operator=cos
  Derivative2 : Derivative
  Integrator : Integrator
  Integrator1 : Integrator
  Integrator2 : Integrator
  M-curve : MATLAB Function  TreatAsAtomicUnit=on
  Multiport Switch : MultiPortSwitch  SaturateOnIntegerOverflow=off  InputSameDT=off
  N-curve : MATLAB Function  TreatAsAtomicUnit=on
  Product : Product
  Product1 : Product
  Product2 : Product
  S-curve : MATLAB Function  TreatAsAtomicUnit=on
  Scope : Scope
  Sin : Trigonometry
  XY Graph : Record  FileSettingsInternal="{\"entries\":[{\"content\":{\"excelSettings\":{\"content\":{},\"type\":\"Streamout.ExcelSettings\"}},\"type\":\"Streamout.FileSettingStorage\",\"uuid\":\"914a34ab-5b3d-44af-9583-0c2c75f12d06\"}],\"packageUris\":[\"http://schema.mathworks.com/mf0/streamout_blocks/R2020a\"],\"version\":\"1.0\"}"  Layout=[1 1]  SignalsInternal="{\"entries\":[{\"content\":{\"signals\":[{\"content\":{\"blockPath\":[\"rlDQNPFC2/Ego Vehicle and Environment3/curvature1/XY Graph\"],\"channel\":[],\"dimensions\":[1],\"domain\":\"rlDQNPFC2/Ego Vehicle and Environment3/curvature1/XY Graph\",\"lineColor\":\"#22b573\",\"plots\":[],\"port\":1,\"sid\":[],\"signalID\":2457,\"signalName\":\"Integrator1\"},\"type\":\"RecordBlkView.Signal\",\"uuid\":\"51aef201-808c-4e46-946c-300a715014d8\"},{\"content\":{\"blockPath\":[\"rlDQNPFC2/Ego Vehicle and Environment3/curvature1/XY Graph\"],\"channel\":[],\"dimensions\":[1],\"domain\":\"rlDQNPFC2/Ego Vehicle and Environment3/curvature1/XY Graph\",\"lineColor\":\"#0072bd\",\"plots\":[],\"port\":2,\"sid\":[],\"signalID\":2460,\"signalName\":\"Integrator2\"},\"type\":\"RecordBlkView.Signal\",\"uuid\":\"bebfd558-065c-412e-a7bd-9710741a958a\"}]},\"type\":\"RecordBlkView.InputSignals\",\"uuid\":\"30e76bc6-5273-4dec-8796-09d7f0daaaf9\"}],\"packageUris\":[\"http://schema.mathworks.com/mf0/streamout_blocks/R2020a\"],\"version\":\"1.0\"}"  VisualizationBindings="{\"xyplotplugin\":{\"info\":[{\"series\":[],\"subplotID\":1}]}}"  CompatibilityTag=XY
  work condition : Constant  Value=target
  curvature : Outport
  wires:
  Integrator1/1 -> XY Graph/1
  Integrator2/1 -> XY Graph/2
  Integrator/1 -> Cos/1, Sin/1
  Derivative2/1 -> Product1/2, Product2/1, Product/2
  Product/1 -> Integrator/1
  Product2/1 -> Integrator2/1
  Sin/1 -> Product2/2
  Product1/1 -> Integrator1/1
  Cos/1 -> Product1/1
  position/1 -> S-curve/1(s), Derivative2/1, M-curve/1(s), N-curve/1(s)
  Multiport Switch/1 -> Product/1, curvature/1, Scope/1
  S-curve/1(rho) -> Multiport Switch/2
  N-curve/1(rho) -> Multiport Switch/3
  work condition/1 -> Multiport Switch/1
  M-curve/1(rho) -> Multiport Switch/4

== system rlDQNPFC2/STEER1/Subsystem ==
  steer : Inport
  e1 : Inport  Port=2
  Compare To Constant1 : simulink/Logic and Bit Operations/Compare To Constant  relop=<  const=0.01  OutDataTypeStr=boolean
  Gain : Gain  Gain=0.1
  Gain2 : Gain  Gain=0.5
  Gain5 : Gain  Gain=2
  Square : Math  Operator=square  SignedPower=on
  Square2 : Math  Operator=square  SignedPower=on
  Sum1 : Sum  Inputs=-++
  Unit Delay : UnitDelay  SampleTime=-1  HasFrameUpgradeWarning=on
  Cost : Outport  VectorParamsAs1DForOutWhenUnconnected=off
  wires:
  e1/1 -> Square/1
  Sum1/1 -> Cost/1
  Gain/1 -> Sum1/2
  steer/1 -> Unit Delay/1
  Square2/1 -> Gain2/1
  Gain2/1 -> Sum1/3
  Unit Delay/1 -> Square2/1
  Compare To Constant1/1 -> Gain5/1
  Square/1 -> Compare To Constant1/1, Gain/1
  Gain5/1 -> Sum1/1

== system rlDQNPFC2/STEER1/Subsystem1 ==
  e1 : Inport
  e2 : Inport  Port=2
  e1dot : Inport  Port=3
  e2dot : Inport  Port=4
  Discrete-Time Integrator : DiscreteIntegrator  SampleTime=-1  ICPrevOutput=DiscIntNeverNeededParam  ICPrevScaledInput=DiscIntNeverNeededParam
  Discrete-Time Integrator1 : DiscreteIntegrator  SampleTime=-1  ICPrevOutput=DiscIntNeverNeededParam  ICPrevScaledInput=DiscIntNeverNeededParam
  Mux : Mux  Inputs=6
  obs : Outport  VectorParamsAs1DForOutWhenUnconnected=off
  wires:
  e1/1 -> Mux/2, Discrete-Time Integrator1/1
  Mux/1 -> obs/1
  Discrete-Time Integrator1/1 -> Mux/1  "integral_error"
  e2/1 -> Mux/4, Discrete-Time Integrator/1
  Discrete-Time Integrator/1 -> Mux/3  "integral_error"
  e1dot/1 -> Mux/5
  e2dot/1 -> Mux/6

== system rlDQNPFC2/STEER2/Subsystem ==
  steer : Inport
  e1 : Inport  Port=2
  Compare To Constant1 : simulink/Logic and Bit Operations/Compare To Constant  relop=<  const=0.01  OutDataTypeStr=boolean
  Gain : Gain  Gain=0.1
  Gain2 : Gain  Gain=0.5
  Gain5 : Gain  Gain=2
  Square : Math  Operator=square  SignedPower=on
  Square2 : Math  Operator=square  SignedPower=on
  Sum1 : Sum  Inputs=-++
  Unit Delay : UnitDelay  SampleTime=-1  HasFrameUpgradeWarning=on
  Cost : Outport  VectorParamsAs1DForOutWhenUnconnected=off
  wires:
  Gain5/1 -> Sum1/1
  Square/1 -> Gain/1, Compare To Constant1/1
  Compare To Constant1/1 -> Gain5/1
  Unit Delay/1 -> Square2/1
  Gain2/1 -> Sum1/3
  Square2/1 -> Gain2/1
  steer/1 -> Unit Delay/1
  Gain/1 -> Sum1/2
  Sum1/1 -> Cost/1
  e1/1 -> Square/1

== system rlDQNPFC2/STEER2/Subsystem1 ==
  e1 : Inport
  e2 : Inport  Port=2
  e1dot : Inport  Port=3
  e2dot : Inport  Port=4
  Discrete-Time Integrator : DiscreteIntegrator  SampleTime=-1  ICPrevOutput=DiscIntNeverNeededParam  ICPrevScaledInput=DiscIntNeverNeededParam
  Discrete-Time Integrator1 : DiscreteIntegrator  SampleTime=-1  ICPrevOutput=DiscIntNeverNeededParam  ICPrevScaledInput=DiscIntNeverNeededParam
  Mux : Mux  Inputs=6
  obs : Outport  VectorParamsAs1DForOutWhenUnconnected=off
  wires:
  e2dot/1 -> Mux/6
  e1dot/1 -> Mux/5
  Discrete-Time Integrator/1 -> Mux/3  "integral_error"
  e2/1 -> Discrete-Time Integrator/1, Mux/4
  Discrete-Time Integrator1/1 -> Mux/1  "integral_error"
  Mux/1 -> obs/1
  e1/1 -> Discrete-Time Integrator1/1, Mux/2

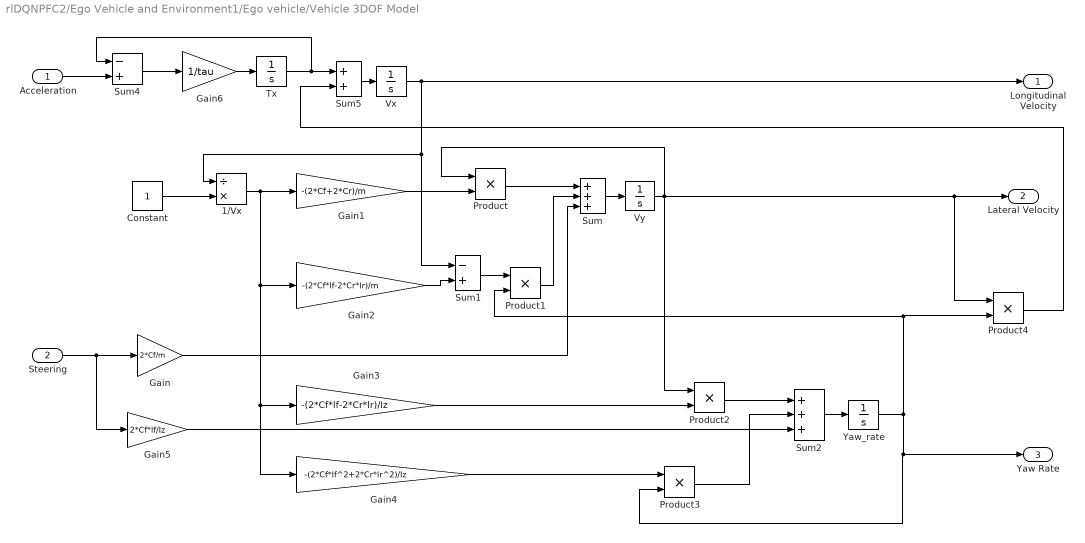
== system rlDQNPFC2/Ego Vehicle and Environment1/Ego vehicle/Vehicle 3DOF Model ==
  Acceleration : Inport
  Steering : Inport  Port=2
  1/Vx : Product  Inputs=/*
  Constant : Constant
  Gain : Gain  Gain=2*Cf/m
  Gain1 : Gain  Gain=-(2*Cf+2*Cr)/m
  Gain2 : Gain  Gain=-(2*Cf*lf-2*Cr*lr)/m
  Gain3 : Gain  Gain=-(2*Cf*lf-2*Cr*lr)/Iz
  Gain4 : Gain  Gain=-(2*Cf*lf^2+2*Cr*lr^2)/Iz
  Gain5 : Gain  Gain=2*Cf*lf/Iz
  Gain6 : Gain  Gain=1/tau
  Product{,1..4} (5 alike) : Product
  Sum : Sum  Inputs=+++
  Sum1 : Sum  Inputs=-+
  Sum2 : Sum  Inputs=+++
  Sum4 : Sum  Inputs=-+
  Sum5 : Sum
  Tx : Integrator
  Vx : Integrator  InitialCondition=v0_FV2
  Vy : Integrator
  "Yaw_rate " : Integrator
  Longitudinal Velocity : Outport  VectorParamsAs1DForOutWhenUnconnected=off
  Lateral Velocity : Outport  Port=2  VectorParamsAs1DForOutWhenUnconnected=off
  Yaw Rate : Outport  Port=3  VectorParamsAs1DForOutWhenUnconnected=off
  wires:
  Vy/1 -> Product/1, Lateral Velocity/1, Product4/1, Product2/1
  Gain2/1 -> Sum1/2
  Product/1 -> Sum/1
  Tx/1 -> Sum5/1, Sum4/1
  Sum/1 -> Vy/1
  "Yaw_rate "/1 -> Yaw Rate/1, Product3/2, Product4/2, Product1/2
  1/Vx/1 -> Gain4/1, Gain3/1, Gain2/1, Gain1/1
  Vx/1 -> 1/Vx/1, Sum1/1, Longitudinal Velocity/1
  Product3/1 -> Sum2/2
  Steering/1 -> Gain/1, Gain5/1
  Acceleration/1 -> Sum4/2
  Sum1/1 -> Product1/1
  Gain/1 -> Sum/3
  Gain1/1 -> Product/2
  Gain6/1 -> Tx/1
  Product2/1 -> Sum2/1
  Sum5/1 -> Vx/1
  Constant/1 -> 1/Vx/2
  Product1/1 -> Sum/2
  Sum4/1 -> Gain6/1
  Gain4/1 -> Product3/1
  Product4/1 -> Sum5/2
  Gain3/1 -> Product2/2
  Gain5/1 -> Sum2/3
  Sum2/1 -> "Yaw_rate "/1

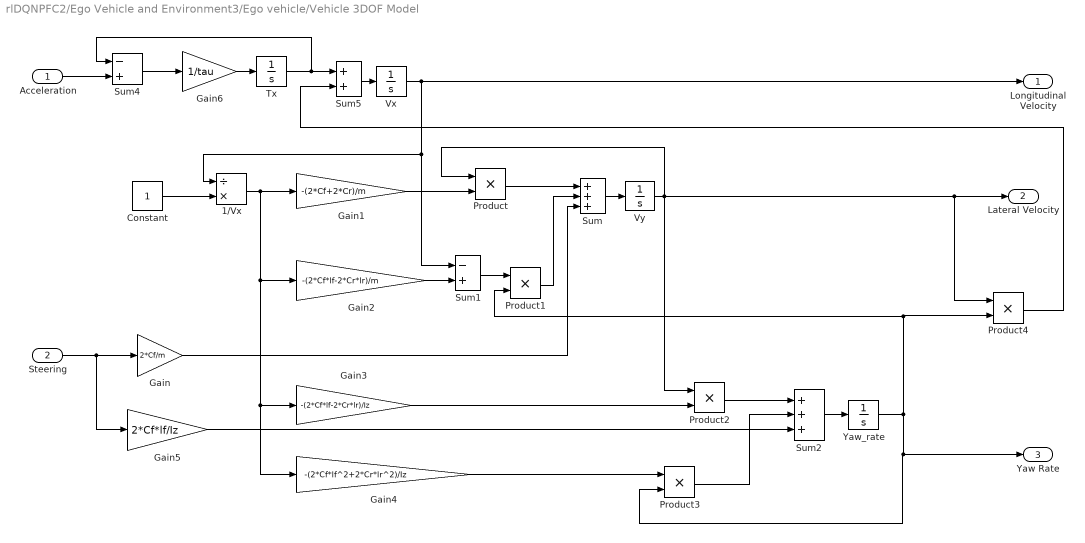
== system rlDQNPFC2/Ego Vehicle and Environment3/Ego vehicle/Vehicle 3DOF Model ==
  Acceleration : Inport
  Steering : Inport  Port=2
  1/Vx : Product  Inputs=/*
  Constant : Constant
  Gain : Gain  Gain=2*Cf/m
  Gain1 : Gain  Gain=-(2*Cf+2*Cr)/m
  Gain2 : Gain  Gain=-(2*Cf*lf-2*Cr*lr)/m
  Gain3 : Gain  Gain=-(2*Cf*lf-2*Cr*lr)/Iz
  Gain4 : Gain  Gain=-(2*Cf*lf^2+2*Cr*lr^2)/Iz
  Gain5 : Gain  Gain=2*Cf*lf/Iz
  Gain6 : Gain  Gain=1/tau
  Product{,1..4} (5 alike) : Product
  Sum : Sum  Inputs=+++
  Sum1 : Sum  Inputs=-+
  Sum2 : Sum  Inputs=+++
  Sum4 : Sum  Inputs=-+
  Sum5 : Sum
  Tx : Integrator
  Vx : Integrator  InitialCondition=v0_FV1
  Vy : Integrator
  "Yaw_rate " : Integrator
  Longitudinal Velocity : Outport  VectorParamsAs1DForOutWhenUnconnected=off
  Lateral Velocity : Outport  Port=2  VectorParamsAs1DForOutWhenUnconnected=off
  Yaw Rate : Outport  Port=3  VectorParamsAs1DForOutWhenUnconnected=off
  wires:
  Vy/1 -> Product/1, Lateral Velocity/1, Product4/1, Product2/1
  Gain2/1 -> Sum1/2
  Product/1 -> Sum/1
  Tx/1 -> Sum5/1, Sum4/1
  Sum/1 -> Vy/1
  "Yaw_rate "/1 -> Yaw Rate/1, Product3/2, Product4/2, Product1/2
  1/Vx/1 -> Gain4/1, Gain3/1, Gain2/1, Gain1/1
  Vx/1 -> 1/Vx/1, Sum1/1, Longitudinal Velocity/1
  Product3/1 -> Sum2/2
  Steering/1 -> Gain/1, Gain5/1
  Acceleration/1 -> Sum4/2
  Sum1/1 -> Product1/1
  Gain/1 -> Sum/3
  Gain1/1 -> Product/2
  Gain6/1 -> Tx/1
  Product2/1 -> Sum2/1
  Sum5/1 -> Vx/1
  Constant/1 -> 1/Vx/2
  Product1/1 -> Sum/2
  Sum4/1 -> Gain6/1
  Gain4/1 -> Product3/1
  Product4/1 -> Sum5/2
  Gain3/1 -> Product2/2
  Gain5/1 -> Sum2/3
  Sum2/1 -> "Yaw_rate "/1

== system rlDQNPFC2/Ego Vehicle and Environment3/Lead vehicle1/ramp1 ==
  note: 工况1：斜坡加速度
  Clock : Clock
  Constant1 : Constant  Value=20
  Constant2 : Constant  Value=40
  Ramp : simulink/Sources/Ramp  slope=0.001  start=0  InitialOutput=0
  Ramp1 : simulink/Sources/Ramp  slope=-0.001  start=20  InitialOutput=0.02
  Ramp2 : simulink/Sources/Ramp  slope=0  start=40  InitialOutput=0
  Relational Operator : RelationalOperator  Operator=<=  OutDataTypeStr=boolean  RndMeth=Simplest  InputSameDT=off
  Relational Operator1 : RelationalOperator  Operator=<=  OutDataTypeStr=boolean  RndMeth=Simplest  InputSameDT=off
  Switch : Switch  Criteria=u2 > Threshold  SaturateOnIntegerOverflow=off  InputSameDT=off
  Switch1 : Switch  Criteria=u2 > Threshold  SaturateOnIntegerOverflow=off  InputSameDT=off
  Out1 : Outport
  wires:
  Constant1/1 -> Relational Operator/2
  Ramp1/1 -> Switch1/1
  Relational Operator/1 -> Switch/2
  Switch1/1 -> Switch/3
  Relational Operator1/1 -> Switch1/2
  Clock/1 -> Relational Operator1/1, Relational Operator/1
  Ramp/1 -> Switch/1
  Constant2/1 -> Relational Operator1/2
  Ramp2/1 -> Switch1/3
  Switch/1 -> Out1/1

== system rlDQNPFC2/Ego Vehicle and Environment3/Lead vehicle1/step1 ==
  note: 工况3：阶梯式加速-减速
  Add : Sum  Inputs=++++
  Step : Step  Time=5  After=0.2  SampleTime=0
  Step1 : Step  Time=8  After=-0.2  SampleTime=0
  Step2 : Step  Time=40  After=-0.2  SampleTime=0
  Step3 : Step  Time=43  After=0.2  SampleTime=0
  a_LV : Outport
  wires:
  Step2/1 -> Add/3
  Step3/1 -> Add/4
  Step/1 -> Add/1
  Add/1 -> a_LV/1  "a_LV"
  Step1/1 -> Add/2

== matlab function rlDQNPFC2/Ego Vehicle and Environment1/curvature1/N-curve ==
  data: s input; rho output
function rho = fcn(s)
% 根据输入s计算输出rho
if s >= 0 && s < 5
  rho = 0;
elseif s >= 5 && s < 10
  rho = 0.025*4;
elseif s >= 10 && s < 30
  rho = -0.025;
elseif s >= 30 && s < 40
  rho = -0.0855;
elseif s >= 40 && s < 60
  rho = 0.057;
else  % s >= 60
  rho = 0;
end

== matlab function rlDQNPFC2/Ego Vehicle and Environment1/curvature1/S-curve ==
  data: s input; rho output
function rho = fcn(s)
% 根据输入s计算输出rho
if s >= 0 && s < 10
  rho = 0;
elseif s >= 10 && s < 40
  rho = 0.005*4;
elseif s >= 40 && s < 70
  rho = -0.005*4;
else  % s >= 70
  rho = 0;
end

== matlab function rlDQNPFC2/Ego Vehicle and Environment3/curvature1/M-curve ==
  data: s input; rho output
function rho = fcn(s)
% 根据输入s计算输出rho
if s >= 0 && s < 5
  rho = 0;
elseif s >= 5 && s < 13
  rho = 0.1;
elseif s >= 13 && s < 25
  rho = -0.0667;
elseif s >= 25 && s < 27
  rho = 0;
elseif s >= 27 && s < 33
  rho = -0.05;
elseif s >= 33 && s < 53
  rho = 0.03;
elseif s >= 53 && s < 59
    rho = -0.05;
elseif s >= 59 && s < 61
    rho = 0;
elseif s >= 61 && s < 73
  rho = -0.0667;
elseif s >= 73 && s < 81
  rho = 0.1;
else  % s >= 70
  rho = 0;
end

== matlab function rlDQNPFC2/Ego Vehicle and Environment3/curvature1/N-curve ==
  data: s input; rho output
function rho = fcn(s)
% 根据输入s计算输出rho
if s >= 0 && s < 5
  rho = 0;
elseif s >= 5 && s < 10
  rho = 0.025*4;
elseif s >= 10 && s < 30
  rho = -0.025;
elseif s >= 30 && s < 40
  rho = -0.0855;
elseif s >= 40 && s < 60
  rho = 0.057;
else  % s >= 60
  rho = 0;
end

== matlab function rlDQNPFC2/Ego Vehicle and Environment3/curvature1/S-curve ==
  data: s input; rho output
function rho = fcn(s)
% 根据输入s计算输出rho
if s >= 0 && s < 10
  rho = 0;
elseif s >= 10 && s < 40
  rho = 0.005*4;
elseif s >= 40 && s < 70
  rho = -0.005*4;
else  % s >= 70
  rho = 0;
end

== matlab function rlDQNPFC2/Ego Vehicle and Environment1/curvature1/M-curve ==
  data: s input; rho output
function rho = fcn(s)
% 根据输入s计算输出rho
if s >= 0 && s < 5
  rho = 0;
elseif s >= 5 && s < 13
  rho = 0.1;
elseif s >= 13 && s < 25
  rho = -0.0667;
elseif s >= 25 && s < 27
  rho = 0;
elseif s >= 27 && s < 33
  rho = -0.05;
elseif s >= 33 && s < 53
  rho = 0.03;
elseif s >= 53 && s < 59
    rho = -0.05;
elseif s >= 59 && s < 61
    rho = 0;
elseif s >= 61 && s < 73
  rho = -0.0667;
elseif s >= 73 && s < 81
  rho = 0.1;
else  % s >= 70
  rho = 0;
end
